simulink model "Zad3"  (R2020b)
settings: Solver=VariableStepAuto  StartTime=0.0  StopTime=0.0  RelTol=1e-3
libraries: CPOiS_SourcesSinks x14, CPOiS_LinearTransforms x12, CPOiS_DataManipulation_DataTypeConversion x12, CPOiS_General x1
settings Model: Creator=Krystian  LastModifiedBy=Krystian

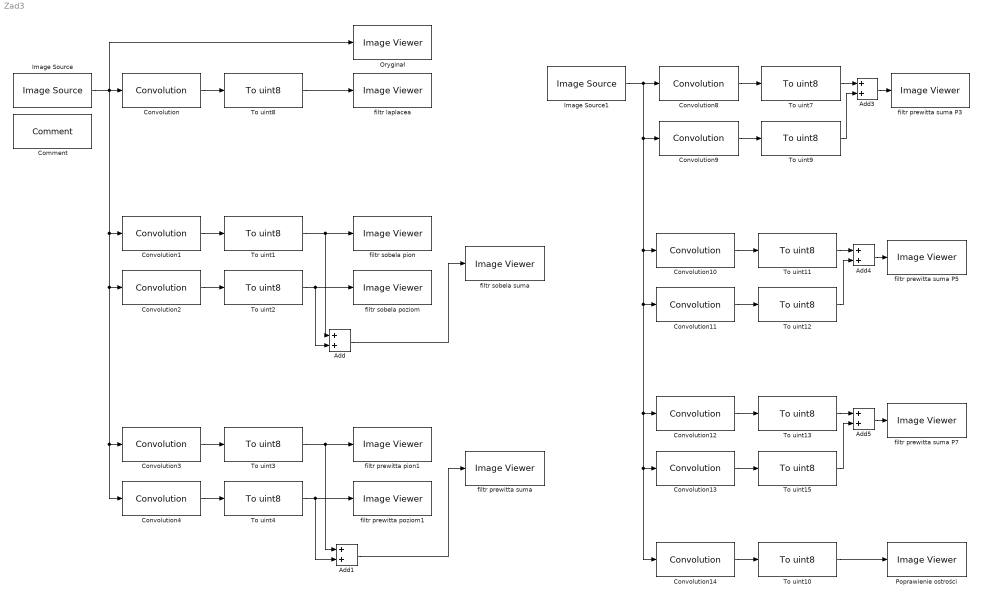
== system Zad3 ==
  Add{,1,3..5} (5 alike) : Sum
  Comment : CPOiS_General/Comment
      settings: SourceProductName=CPOiS - Digital image and signal processing
  Convolution : CPOiS_LinearTransforms/Convolution  ConvolutionMatrix=[1,1,1;1,-8,1;1,1,1]
      settings: SourceProductName=CPOiS - Digital image and signal processing
  Convolution1 : CPOiS_LinearTransforms/Convolution  ConvolutionMatrix=[-1,0,1;-2,0,2;-1,0,1]
      settings: SourceProductName=CPOiS - Digital image and signal processing
  Convolution10 : CPOiS_LinearTransforms/Convolution  ConvolutionMatrix=[-1,-2,0,2,1;-1,-2,0,2,1;-1,-2,0,2,1;-1,-2,0,2,1;-1,-2,0,2,1]
      settings: SourceProductName=CPOiS - Digital image and signal processing
  Convolution11 : CPOiS_LinearTransforms/Convolution  ConvolutionMatrix=[-1,-1,-1,-1,-1;-2,-2,-2,-2,-2;0,0,0,0,0;2,2,2,2,2; 1,1,1,1,1]
      settings: SourceProductName=CPOiS - Digital image and signal processing
  Convolution12 : CPOiS_LinearTransforms/Convolution  ConvolutionMatrix=[-1,-4,-5,0,5,4,1;-1,-4,-5,0,5,4,1;-1,-4,-5,0,5,4,1;-1,-4,-5,0,5,4,1;-1,-4,-5,0,5,4,1;-1,-4,-5,0,5,4,1;-1,-4,-5,0,5,4,1]
      settings: SourceProductName=CPOiS - Digital image and signal processing
  Convolution13 : CPOiS_LinearTransforms/Convolution  ConvolutionMatrix=[-1,-1,-1,-1,-1,-1,-1;-4,-4,-4,-4,-4,-4,-4;-5,-5,-5,-5,-5,-5,-5;0,0,0,0,0,0,0;5,5,5,5,5,5,5;4,4,4,4,4,4,4;1,1,1,1,1,1,1]
      settings: SourceProductName=CPOiS - Digital image and signal processing
  Convolution14 : CPOiS_LinearTransforms/Convolution  ConvolutionMatrix=[0,-1,0;-1,5,-1;0,-1,0]
      settings: SourceProductName=CPOiS - Digital image and signal processing
  Convolution2 : CPOiS_LinearTransforms/Convolution  ConvolutionMatrix=[-1,-2,-1;0,0,0;1,2,1]
      settings: SourceProductName=CPOiS - Digital image and signal processing
  Convolution3 : CPOiS_LinearTransforms/Convolution  ConvolutionMatrix=[-1,0,1;-1,0,1;-1,0,1]
      settings: SourceProductName=CPOiS - Digital image and signal processing
  Convolution4 : CPOiS_LinearTransforms/Convolution  ConvolutionMatrix=[-1,-1,-1;0,0,0;1,1,1]
      settings: SourceProductName=CPOiS - Digital image and signal processing
  Convolution8 : CPOiS_LinearTransforms/Convolution  ConvolutionMatrix=[-1,0,1;-1,0,1;-1,0,1]
      settings: SourceProductName=CPOiS - Digital image and signal processing
  Convolution9 : CPOiS_LinearTransforms/Convolution  ConvolutionMatrix=[-1,-1,-1;0,0,0;1,1,1]
      settings: SourceProductName=CPOiS - Digital image and signal processing
  Image Source : CPOiS_SourcesSinks/Image Source  FileSelection=cameraman.tif
      settings: SourceProductName=CPOiS - Digital image and signal processing
  Image Source1 : CPOiS_SourcesSinks/Image Source  FileSelection=cameraman.tif
      settings: SourceProductName=CPOiS - Digital image and signal processing
  Oryginał : CPOiS_SourcesSinks/Image Viewer
      settings: SourceProductName=CPOiS - Digital image and signal processing
  Poprawienie ostrości : CPOiS_SourcesSinks/Image Viewer
      settings: SourceProductName=CPOiS - Digital image and signal processing
  To uint{1..4,7..13,15} (12 alike) : CPOiS_DataManipulation_DataTypeConversion/To uint8
      settings: SourceProductName=CPOiS - Digital image and signal processing
  "filtr laplacea " : CPOiS_SourcesSinks/Image Viewer
      settings: SourceProductName=CPOiS - Digital image and signal processing
  filtr prewitta pion1 : CPOiS_SourcesSinks/Image Viewer
      settings: SourceProductName=CPOiS - Digital image and signal processing
  filtr prewitta poziom1 : CPOiS_SourcesSinks/Image Viewer
      settings: SourceProductName=CPOiS - Digital image and signal processing
  filtr prewitta suma : CPOiS_SourcesSinks/Image Viewer
      settings: SourceProductName=CPOiS - Digital image and signal processing
  filtr prewitta suma P3 : CPOiS_SourcesSinks/Image Viewer
      settings: SourceProductName=CPOiS - Digital image and signal processing
  filtr prewitta suma P5 : CPOiS_SourcesSinks/Image Viewer
      settings: SourceProductName=CPOiS - Digital image and signal processing
  filtr prewitta suma P7 : CPOiS_SourcesSinks/Image Viewer
      settings: SourceProductName=CPOiS - Digital image and signal processing
  filtr sobela pion : CPOiS_SourcesSinks/Image Viewer
      settings: SourceProductName=CPOiS - Digital image and signal processing
  filtr sobela poziom : CPOiS_SourcesSinks/Image Viewer
      settings: SourceProductName=CPOiS - Digital image and signal processing
  filtr sobela suma : CPOiS_SourcesSinks/Image Viewer
      settings: SourceProductName=CPOiS - Digital image and signal processing
  wires:
  Convolution3/1 -> To uint3/1
  To uint3/1 -> filtr prewitta pion1/1, Add1/1
  Convolution4/1 -> To uint4/1
  Add1/1 -> filtr prewitta suma/1
  To uint4/1 -> Add1/2, filtr prewitta poziom1/1
  Add/1 -> filtr sobela suma/1
  Convolution2/1 -> To uint2/1
  To uint8/1 -> "filtr laplacea "/1
  To uint2/1 -> Add/2, filtr sobela poziom/1
  Convolution1/1 -> To uint1/1
  To uint1/1 -> filtr sobela pion/1, Add/1
  Convolution/1 -> To uint8/1
  Image Source/1 -> Convolution1/1, Convolution2/1, Convolution3/1, Convolution4/1, Convolution/1, Oryginał/1
  Add3/1 -> filtr prewitta suma P3/1
  Convolution11/1 -> To uint12/1
  To uint15/1 -> Add5/2
  To uint11/1 -> Add4/1
  Convolution10/1 -> To uint11/1
  Convolution12/1 -> To uint13/1
  Image Source1/1 -> Convolution12/1, Convolution13/1, Convolution14/1, Convolution11/1, Convolution10/1, Convolution9/1, Convolution8/1
  Convolution14/1 -> To uint10/1
  To uint9/1 -> Add3/2
  To uint13/1 -> Add5/1
  Add5/1 -> filtr prewitta suma P7/1
  Convolution9/1 -> To uint9/1
  To uint12/1 -> Add4/2
  Convolution8/1 -> To uint7/1
  To uint7/1 -> Add3/1
  Convolution13/1 -> To uint15/1
  Add4/1 -> filtr prewitta suma P5/1
  To uint10/1 -> Poprawienie ostrości/1
